simulink model "Control_Loop4_2Model"  (R2013b)
settings: Solver=ode45  StartTime=0.0  StopTime=200  RelTol=1e-3
libraries: commutil2 x756, xpclib x100, etargetslib x98, dspnetwork x98, powerlib_meascontrol x24, commcrc2 x14, dspadpt3 x4, simulink_extras x4, dspmtrx3 x4, simulink x1
(part 1 of 7)
settings Model: Creator=HESL  LastModifiedBy=ANKITA003

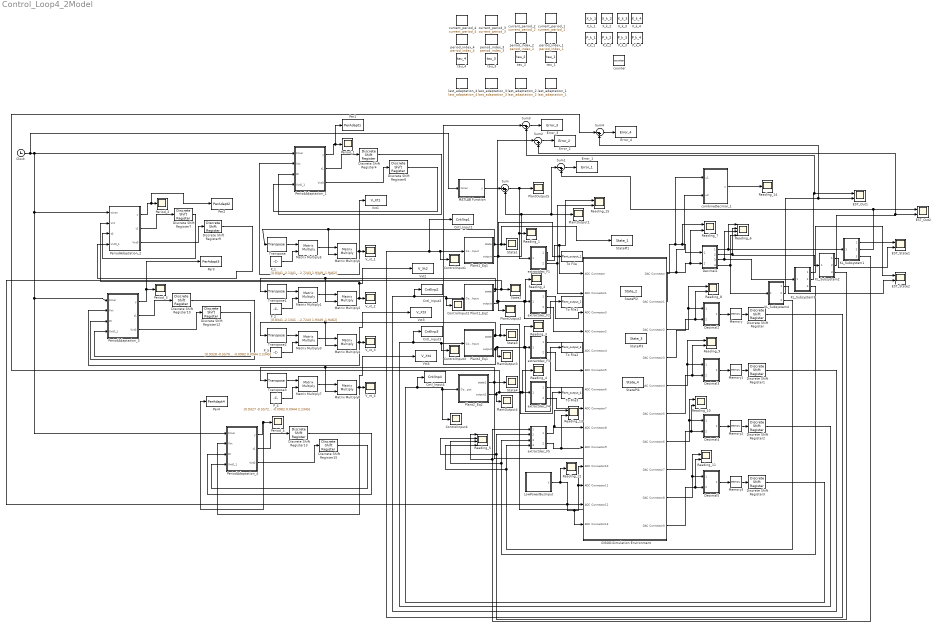
== system Control_Loop4_2Model ==
  Clock : Clock
  Cntl_Input1 : ToFile  Filename=CntlInp1  MatrixName=u
  Cntl_Input2 : ToFile  Filename=CntlInp2  MatrixName=u
  Cntl_Input3 : ToFile  Filename=CntlInp3  MatrixName=u
  Cntl_Input4 : ToFile  Filename=CntlInp4  MatrixName=u
  ControlInput{1..4} (4 alike) : Scope
      ControlInput1 settings: YMin=-4.25  YMax=1.25
      ControlInput2 settings: YMin=-9  YMax=0
      ControlInput3 settings: YMin=-1.60965  YMax=-1.45635  SaveName=ScopeData6
      ControlInput4 settings: YMin=0.01045  YMax=0.01155  SaveName=ScopeData9
  Decimal1 : Subsystem
  Decimal2 : Subsystem
  Decimal3 : Subsystem
  Decimal4 : Subsystem
  Decimal5 : Subsystem
  Discrete Shift Register : powerlib_meascontrol/Additional Components/Discrete Shift Register  NSamples=1  InitialValue=0  Ts=0.150
  Discrete Shift Register1 : powerlib_meascontrol/Additional Components/Discrete Shift Register  NSamples=1  InitialValue=0  Ts=0.150
  Discrete Shift Register{4,6..7,9..10,12..13,15} (8 alike) : powerlib_meascontrol/Additional Components/Discrete Shift Register  NSamples=1  InitialValue=0  Ts=1
  Discrete Shift Register2 : powerlib_meascontrol/Additional Components/Discrete Shift Register  NSamples=1  InitialValue=0  Ts=0.225
  Discrete Shift Register3 : powerlib_meascontrol/Additional Components/Discrete Shift Register  NSamples=1  InitialValue=0  Ts=0.225
  EST_Out1 : Scope  NumInputPorts=2
      settings: YMin=-1.975~-1.92  YMax=-1.55~-1.77  SaveName=ScopeData15
  EST_Out2 : Scope  NumInputPorts=2
      settings: YMin=-4.75e-05~1.71875  YMax=-1e-05~1.71905  SaveName=ScopeData16
  EST_State1 : Scope  NumInputPorts=2
      settings: YMin=-35~-0.1  YMax=40~1.9  SaveName=ScopeData13
  EST_State2 : Scope  NumInputPorts=2
      settings: YMin=-2.5~-0.0003  YMax=1.5~0.001  SaveName=ScopeData14
  Error_1 : ToFile  Filename=Error_1  MatrixName=err_1
  Error_2 : ToFile  Filename=Error_2  MatrixName=err_1
  Error_3 : ToFile  Filename=Error_3  MatrixName=err_1
  Error_4 : ToFile  Filename=Error_4  MatrixName=err_1
  GISOO-Simulation Environment : Subsystem  TreatAsAtomicUnit=on
  KL_Subsystem1 : Subsystem
  KL_Subsystem2 : Subsystem
  KL_Subsystem3 : Subsystem
  KL_Subsystem4 : Subsystem
  LowPowerBusInput : MATLAB Function  TreatAsAtomicUnit=on  SystemSampleTime=0.200
  MATLAB Function : MATLAB Function  TreatAsAtomicUnit=on  SystemSampleTime=0.010
  Matrix Multiply1 : Product  Multiplication=Matrix(*)  SampleTime=0.150
  Matrix Multiply2 : Product  Multiplication=Matrix(*)  SampleTime=0.150
  Matrix Multiply{3..4,7..8} (4 alike) : Product  Multiplication=Matrix(*)  SampleTime=0.225
  Matrix Multiply5 : Product  Multiplication=Matrix(*)  SampleTime=1
  Matrix Multiply6 : Product  Multiplication=Matrix(*)  SampleTime=1
  Memory{,1..3} (4 alike) : Memory
  P_1 : Constant  Value=[0.8341 -2.1341 0.2898 -0.9410;-2.1341 -25.1720 3.5962 -12.7243;0.2898 3.5962 0.5577 1.9349;-0.9410 -12.7243 1.9349 -1.9462]  VectorParams1D=off  SampleTime=1
  P_2 : Constant  Value=[0.8341 -2.1341 0.2898 -0.9410;-2.1341 -25.1720 3.5962 -12.7243;0.2898 3.5962 0.5577 1.9349;-0.9410 -12.7243 1.9349 -1.9462]  VectorParams1D=off  SampleTime=0.150
  P_3 : Constant  Value=[0.9328 -0.5570 0.0394 0.0140;-0.5570 -2.3354 0.2168 -0.0982;0.0394 0.2168 1.0331 0.0944;0.0140 -0.0982 0.0944 2.2345]  VectorParams1D=off  SampleTime=0.225
  P_4 : Constant  Value=[0.9327 -0.5572 0.0394 0.0140;-0.5572 -2.3356 0.2168 -0.0982;0.0394 0.2168 1.0331 0.0944;0.0140 -0.0982 0.0944 2.2345]  VectorParams1D=off  SampleTime=0.225
  P_k_1 : DataStoreMemory  DataStoreName=P_k_1  InitialValue=10*eye(4)  OutDataTypeStr=double
  P_k_2 : DataStoreMemory  DataStoreName=P_k_2  InitialValue=10*eye(4)  OutDataTypeStr=double
  P_k_3 : DataStoreMemory  DataStoreName=P_k_3  InitialValue=10*eye(4)  OutDataTypeStr=double
  P_k_4 : DataStoreMemory  DataStoreName=P_k_4  InitialValue=10*eye(4)  OutDataTypeStr=double
  Per1 : ToFile  Filename=PerAdapt1  MatrixName=P1
  Per2 : ToFile  Filename=PerAdapt2  MatrixName=P2
  Per3 : ToFile  Filename=PerAdapt3  MatrixName=P3
  Per4 : ToFile  Filename=PerAdapt4  MatrixName=P4
  PeriodAdaptation_1 : MATLAB Function  RequirementInfo={} %GIDa_850bbe14_d9da_4034_8937_a8dbb2f822c9  TreatAsAtomicUnit=on  SystemSampleTime=1
  PeriodAdaptation_2 : MATLAB Function  RequirementInfo={} %GIDa_a70684f9_3044_4532_9a1c_a31c50b95e8e  TreatAsAtomicUnit=on  SystemSampleTime=1
  PeriodAdaptation_3 : MATLAB Function  RequirementInfo={} %GIDa_89bb9df0_2bef_4001_9282_b413ac28a927  TreatAsAtomicUnit=on  SystemSampleTime=1
  PeriodAdaptation_4 : MATLAB Function  RequirementInfo={} %GIDa_da02a095_aa0b_4737_8edc_96c2e4425495  TreatAsAtomicUnit=on  SystemSampleTime=1
  Period_{1..4} (4 alike) : Scope
      Period_1 settings: TickLabels=on  YMin=19  YMax=21  SaveName=ScopeData21  SampleInput=on
      Period_2 settings: TickLabels=on  YMin=57  YMax=63  SaveName=ScopeData22  SampleInput=on
      Period_3 settings: TickLabels=on  YMin=15  YMax=15  SaveName=ScopeData23  SampleInput=on
      Period_4 settings: TickLabels=on  YMin=15  YMax=15  SaveName=ScopeData24  SampleInput=on
  Plant1_Eq1 : Subsystem
  Plant1_Eq2 : Subsystem
  Plant2_Eq1 : Subsystem
  Plant2_Eq2 : Subsystem
  PlantOutput{1..5} (5 alike) : Scope
      PlantOutput1 settings: YMin=0.097  YMax=0.117  SaveName=ScopeData4
      PlantOutput2 settings: TimeRange=200  YMin=1.71906  YMax=1.71906  SaveName=ScopeData2
      PlantOutput3 settings: TimeRange=200  YMin=1.7729  YMax=1.7729  SaveName=ScopeData7
      PlantOutput4 settings: YMin=-0.835427  YMax=-0.835427  SaveName=ScopeData10
      PlantOutput5 settings: TimeRange=200  YMin=1.72358  YMax=1.905  SaveName=ScopeData39
  Reading_{1..4,12,14} (6 alike) : Scope
      Reading_1 settings: YMin=1.71875  YMax=1.71935  SaveName=ScopeData25
      Reading_12 settings: YMin=20  YMax=20  SaveName=ScopeData36
      Reading_14 settings: YMin=0  YMax=1.75  SaveName=ScopeData38
      Reading_2 settings: YMin=1.72358  YMax=1.905  SaveName=ScopeData26
      Reading_3 settings: YMin=1.41328  YMax=1.56204  SaveName=ScopeData27
      Reading_4 settings: YMin=1.41328  YMax=1.56204  SaveName=ScopeData28
  Reading_{7..11,13,15} (7 alike) : Scope  NumInputPorts=2
      Reading_10 settings: YMin=1001~2533  YMax=1001~2533  SaveName=ScopeData34
      Reading_11 settings: YMin=1001~3533  YMax=1001~3533  SaveName=ScopeData35
      Reading_13 settings: YMin=1001~0  YMax=1003~3750  SaveName=ScopeData37
      Reading_15 settings: YMin=1~719.057  YMax=1~719.057  SaveName=ScopeData40
      Reading_7 settings: YMin=1~500  YMax=1~4000  SaveName=ScopeData31
      Reading_8 settings: YMin=1003~260  YMax=1003~440  SaveName=ScopeData32
      Reading_9 settings: YMin=950~1187.5  YMax=1050~1312.5  SaveName=ScopeData33
  Reading_5 : Scope  NumInputPorts=4
      settings: YMin=-3.3425~-3.3425~-1.61025~-1.61025  YMax=-3.3225~-3.3225~-1.45689~-1.45689  SaveName=ScopeData29  MaxDataPoints=100000
  Reading_6 : Scope  NumInputPorts=4
      settings: YMin=1.718~1.718~1.4459~1.4459  YMax=1.719~1.719~1.5981~1.5981  SaveName=ScopeData30  MaxDataPoints=100000
  State{1..4} (4 alike) : Scope
      State1 settings: YMin=-0.5  YMax=8  SaveName=ScopeData5
      State2 settings: YMin=0.4  YMax=1  SaveName=ScopeData3
      State3 settings: YMin=0.15  YMax=1.05  SaveName=ScopeData8
      State4 settings: YMin=-0.055  YMax=-0.042  SaveName=ScopeData12
  StatePl1 : ToFile  Filename=State_1  MatrixName=x
  StatePl2 : ToFile  Filename=State_2  MatrixName=x
  StatePl3 : ToFile  Filename=State_3  MatrixName=x
  StatePl4 : ToFile  Filename=State_4  MatrixName=x
  Sum : Sum  Inputs=|++
  Sum{1..4} (4 alike) : Sum  Inputs=|-+  SampleTime=1
  To File : ToFile  Filename=Plant_output_1  MatrixName=Out
  To File1 : ToFile  Filename=Plant_output_2  MatrixName=Out
  To File2 : ToFile  Filename=Plant_output_3  MatrixName=Out
  To File3 : ToFile  Filename=Plant_output_4  MatrixName=Out
  Transpose{,1..3} (4 alike) : dspmtrx3/Transpose  Hermitian=off  overflowFlag=off
  V_xt_{1..4} (4 alike) : Scope
      V_xt_1 settings: TickLabels=on  YMin=-0.19  YMax=-0.085  SaveName=ScopeData17  SampleInput=on
      V_xt_2 settings: TickLabels=on  YMin=-2.5e-06  YMax=4.5e-05  SaveName=ScopeData18  SampleInput=on
      V_xt_3 settings: TickLabels=on  YMin=0.0031225  YMax=0.003133  SaveName=ScopeData19  SampleInput=on
      V_xt_4 settings: TickLabels=on  YMin=0.00322  YMax=0.00322002  SaveName=ScopeData20  SampleInput=on
  Vxt1 : ToFile  Filename=V_Xt1  MatrixName=Vxt
  Vxt2 : ToFile  Filename=V_Xt2  MatrixName=Vxt
  Vxt3 : ToFile  Filename=V_Xt3  MatrixName=Vxt
  Vxt4 : ToFile  Filename=V_Xt4  MatrixName=Vxt
  X_k_1 : DataStoreMemory  DataStoreName=X_k_1  InitialValue=zeros(4,1)  OutDataTypeStr=double
  X_k_2 : DataStoreMemory  DataStoreName=X_k_2  InitialValue=zeros(4,1)  OutDataTypeStr=double
  X_k_3 : DataStoreMemory  DataStoreName=X_k_3  InitialValue=zeros(4,1)  OutDataTypeStr=double
  X_k_4 : DataStoreMemory  DataStoreName=X_k_4  InitialValue=zeros(4,1)  OutDataTypeStr=double
  combineDecimal_1 : MATLAB Function  TreatAsAtomicUnit=on  SystemSampleTime=0.010
  counter : DataStoreMemory  DataStoreName=counter  OutDataTypeStr=double
  current_period_1 : DataStoreMemory  DataStoreName=current_period_1  InitialValue=10  OutDataTypeStr=double
  current_period_2 : DataStoreMemory  DataStoreName=current_period_2  InitialValue=10  OutDataTypeStr=double
  current_period_3 : DataStoreMemory  DataStoreName=current_period_3  InitialValue=15  OutDataTypeStr=double
  current_period_4 : DataStoreMemory  DataStoreName=current_period_4  InitialValue=15  OutDataTypeStr=double
  extractdec_F1 : Subsystem
  extractdec_F2 : Subsystem
  extractdec_F3 : Subsystem
  extractdec_F4 : Subsystem
  extractdec_F5 : Subsystem
  last_adaptation_1 : DataStoreMemory  DataStoreName=last_adaptation_1  OutDataTypeStr=double
  last_adaptation_2 : DataStoreMemory  DataStoreName=last_adaptation_2  OutDataTypeStr=double
  last_adaptation_3 : DataStoreMemory  DataStoreName=last_adaptation_3  OutDataTypeStr=double
  last_adaptation_4 : DataStoreMemory  DataStoreName=last_adaptation_4  OutDataTypeStr=double
  period_index_1 : DataStoreMemory  DataStoreName=period_index_1  InitialValue=1  OutDataTypeStr=double
  period_index_2 : DataStoreMemory  DataStoreName=period_index_2  InitialValue=1  OutDataTypeStr=double
  period_index_3 : DataStoreMemory  DataStoreName=period_index_3  InitialValue=1  OutDataTypeStr=double
  period_index_4 : DataStoreMemory  DataStoreName=period_index_4  InitialValue=1  OutDataTypeStr=double
  tau_1 : DataStoreMemory  DataStoreName=tau_1  OutDataTypeStr=double
  tau_2 : DataStoreMemory  DataStoreName=tau_2  OutDataTypeStr=double
  tau_3 : DataStoreMemory  DataStoreName=tau_3  OutDataTypeStr=double
  tau_4 : DataStoreMemory  DataStoreName=tau_4  OutDataTypeStr=double
  wires:
  Plant2_Eq1/2(output) -> To File2/1, extractdec_F3/1(In1), Reading_3/1, PlantOutput3/1, Sum3/1
  extractdec_F1/1(Out1) -> Reading_15/1, GISOO-Simulation Environment/1(ADC Connector)
  extractdec_F1/2(Out2) -> GISOO-Simulation Environment/2(ADC Connector1), Reading_15/2
  extractdec_F2/1(Out1) -> GISOO-Simulation Environment/3(ADC Connector3)
  extractdec_F2/2(Out2) -> GISOO-Simulation Environment/4(ADC Connector2)
  extractdec_F3/1(Out1) -> GISOO-Simulation Environment/5(ADC Connector4)
  extractdec_F3/2(Out2) -> GISOO-Simulation Environment/6(ADC Connector5)
  extractdec_F4/1(Out1) -> GISOO-Simulation Environment/7(ADC Connector6)
  extractdec_F4/2(Out2) -> GISOO-Simulation Environment/8(ADC Connector7)
  extractdec_F5/1(Out1) -> Reading_13/1, GISOO-Simulation Environment/9(ADC Connector8)
  extractdec_F5/2(Out2) -> Reading_13/2, GISOO-Simulation Environment/10(ADC Connector9)
  LowPowerBusInput/1(y) -> Reading_12/1, GISOO-Simulation Environment/14(ADC Connector13), GISOO-Simulation Environment/11(ADC Connector10), GISOO-Simulation Environment/12(ADC Connector11), GISOO-Simulation Environment/13(ADC Connector12)
  GISOO-Simulation Environment/1(DAC Connector) -> combineDecimal_1/1(u1), Reading_7/1, Decimal1/1(In1)
  GISOO-Simulation Environment/4(DAC Connector3) -> Reading_8/2, Decimal2/2(In2)
  GISOO-Simulation Environment/3(DAC Connector2) -> Reading_8/1, Decimal2/1(In1)
  GISOO-Simulation Environment/5(DAC Connector4) -> Reading_9/1, Decimal3/1(In1)
  GISOO-Simulation Environment/6(DAC Connector5) -> Reading_9/2, Decimal3/2(In2)
  GISOO-Simulation Environment/7(DAC Connector6) -> Reading_10/1, Decimal4/1(In1)
  GISOO-Simulation Environment/8(DAC Connector7) -> Reading_10/2, Decimal4/2(In2)
  GISOO-Simulation Environment/9(DAC Connector8) -> Reading_11/1, Decimal5/1(In1)
  GISOO-Simulation Environment/10(DAC Connector9) -> Reading_11/2, Decimal5/2(In2)
  Decimal1/1(Out1) -> KL_Subsystem1/1(In1), Reading_6/1
  Decimal1/2(Out2) -> KL_Subsystem2/1(In1), Reading_6/2
  Decimal1/3(Out3) -> Reading_6/3, KL_Subsystem3/1(In1)
  Decimal1/4(Out4) -> KL_Subsystem4/1(In1), Reading_6/4
  Discrete Shift Register/1 -> Cntl_Input1/1, Plant1_Eq1/1(ControlInput), ControlInput1/1
  Discrete Shift Register1/1 -> Cntl_Input2/1, ControlInput2/1, Plant1_Eq2/1(ControlInput)
  Discrete Shift Register2/1 -> ControlInput3/1, Plant2_Eq1/1(ControlInput), Cntl_Input3/1
  Decimal2/1(Out1) -> Memory/1
  Memory/1 -> Discrete Shift Register/1
  Decimal3/1(Out1) -> Memory1/1
  Memory1/1 -> Discrete Shift Register1/1
  Decimal4/1(Out1) -> Memory2/1
  Memory2/1 -> Discrete Shift Register2/1
  Decimal5/1(Out1) -> Memory3/1
  Memory3/1 -> Discrete Shift Register3/1
  KL_Subsystem1/3(Out3) -> Reading_5/1, extractdec_F5/1(In1)
  KL_Subsystem2/3(Out3) -> Reading_5/2, extractdec_F5/2(In2)
  KL_Subsystem3/3(Out3) -> Reading_5/3, extractdec_F5/3(In3)
  KL_Subsystem4/3(Out3) -> Reading_5/4, extractdec_F5/4(In4)
  KL_Subsystem1/1(Out1) -> EST_State1/1
  KL_Subsystem2/1(Out1) -> EST_State1/2
  KL_Subsystem3/1(Out1) -> EST_State2/1
  KL_Subsystem4/1(Out1) -> EST_State2/2
  KL_Subsystem4/2(Out2) -> EST_Out1/2, Sum4/2
  Transpose/1 -> Matrix Multiply5/1
  Matrix Multiply5/1 -> Matrix Multiply6/1
  P_1/1 -> Matrix Multiply5/2
  Plant1_Eq1/1(state) -> Matrix Multiply6/2, Transpose/1, StatePl1/1, State1/1
  Transpose1/1 -> Matrix Multiply1/1
  Matrix Multiply1/1 -> Matrix Multiply2/1
  P_2/1 -> Matrix Multiply1/2
  Plant1_Eq2/1(state) -> Matrix Multiply2/2, Transpose1/1, StatePl2/1, State2/1
  Transpose2/1 -> Matrix Multiply3/1
  Matrix Multiply3/1 -> Matrix Multiply4/1
  P_3/1 -> Matrix Multiply3/2
  Plant2_Eq1/1(state) -> Matrix Multiply4/2, Transpose2/1, StatePl3/1, State3/1
  Transpose3/1 -> Matrix Multiply7/1
  Matrix Multiply7/1 -> Matrix Multiply8/1
  P_4/1 -> Matrix Multiply7/2
  Plant2_Eq2/1(state1) -> StatePl4/1, State4/1, Matrix Multiply8/2, Transpose3/1
  Matrix Multiply6/1 -> Vxt1/1, PeriodAdaptation_1/2(Vxt), V_xt_1/1
  PeriodAdaptation_1/2(t1) -> Discrete Shift Register4/1
  Discrete Shift Register4/1 -> PeriodAdaptation_1/3(t0)
  PeriodAdaptation_1/3(Vxt0) -> Discrete Shift Register6/1
  Discrete Shift Register6/1 -> PeriodAdaptation_1/4(Vxt0_1)
  PeriodAdaptation_1/1(y) -> Per1/1, Period_1/1
  Matrix Multiply2/1 -> Vxt2/1, PeriodAdaptation_2/2(Vxt), V_xt_2/1
  PeriodAdaptation_2/2(t1) -> Discrete Shift Register7/1
  Discrete Shift Register7/1 -> PeriodAdaptation_2/3(t0)
  PeriodAdaptation_2/3(Vxt0) -> Discrete Shift Register9/1
  Discrete Shift Register9/1 -> PeriodAdaptation_2/4(Vxt0_1)
  PeriodAdaptation_2/1(y) -> Per2/1, Period_2/1
  Matrix Multiply4/1 -> PeriodAdaptation_3/2(Vxt), Vxt3/1, V_xt_3/1
  PeriodAdaptation_3/2(t1) -> Discrete Shift Register10/1
  Discrete Shift Register10/1 -> PeriodAdaptation_3/3(t0)
  PeriodAdaptation_3/3(Vxt0) -> Discrete Shift Register12/1
  Discrete Shift Register12/1 -> PeriodAdaptation_3/4(Vxt0_1)
  PeriodAdaptation_3/1(y) -> Per3/1, Period_3/1
  Matrix Multiply8/1 -> PeriodAdaptation_4/2(Vxt), Vxt4/1, V_xt_4/1
  PeriodAdaptation_4/2(t1) -> Discrete Shift Register13/1
  Discrete Shift Register13/1 -> PeriodAdaptation_4/3(t0)
  PeriodAdaptation_4/3(Vxt0) -> Discrete Shift Register15/1
  Discrete Shift Register15/1 -> PeriodAdaptation_4/4(Vxt0_1)
  PeriodAdaptation_4/1(y) -> Per4/1, Period_4/1
  Clock/1 -> MATLAB Function/1(timer), PeriodAdaptation_4/1(timer), PeriodAdaptation_3/1(timer), PeriodAdaptation_2/1(timer), PeriodAdaptation_1/1(timer)
  Plant1_Eq1/2(output) -> To File/1, Sum1/1, PlantOutput1/1, Sum/2
  GISOO-Simulation Environment/2(DAC Connector1) -> combineDecimal_1/2(u2), Reading_7/2, Decimal1/2(In2)
  combineDecimal_1/1(y) -> Reading_14/1
  MATLAB Function/1(y) -> Sum/1
  Sum/1 -> Reading_1/1, extractdec_F1/1(In1), PlantOutput5/1
  KL_Subsystem1/2(Out2) -> Sum1/2, EST_Out2/1
  Sum1/1 -> Error_1/1
  Sum2/1 -> Error_2/1
  Sum3/1 -> Error_3/1
  Sum4/1 -> Error_4/1
  Plant1_Eq2/2(output) -> To File1/1, Reading_2/1, extractdec_F2/1(In1), PlantOutput2/1, Sum2/1
  KL_Subsystem2/2(Out2) -> EST_Out2/2, Sum2/2
  KL_Subsystem3/2(Out2) -> EST_Out1/1, Sum3/2
  Plant2_Eq2/2(output1) -> PlantOutput4/1, Sum4/1, To File3/1, Reading_4/1, extractdec_F4/1(In1)
  Discrete Shift Register3/1 -> Cntl_Input4/1, ControlInput4/1, Plant2_Eq2/1(ControlInput)

== system Control_Loop4_2Model/Decimal1 ==
  In1 : Inport
  In2 : Inport  Port=2
  Discrete Shift Register{,1..3} (4 alike) : powerlib_meascontrol/Additional Components/Discrete Shift Register  NSamples=1  InitialValue=0  Ts=0.010
  combineDecimal_1 : MATLAB Function  TreatAsAtomicUnit=on  SystemSampleTime=0.010
  Out1 : Outport
  Out2 : Outport  Port=2
  Out3 : Outport  Port=3
  Out4 : Outport  Port=4
  wires:
  combineDecimal_1/1(y1) -> Out1/1
  In2/1 -> combineDecimal_1/2(u2)
  In1/1 -> combineDecimal_1/1(u1)
  combineDecimal_1/5(x1) -> Discrete Shift Register/1
  combineDecimal_1/6(x2) -> Discrete Shift Register1/1
  combineDecimal_1/7(x3) -> Discrete Shift Register2/1
  combineDecimal_1/8(x4) -> Discrete Shift Register3/1
  Discrete Shift Register3/1 -> combineDecimal_1/6(x4_prev)
  Discrete Shift Register2/1 -> combineDecimal_1/5(x3_prev)
  Discrete Shift Register1/1 -> combineDecimal_1/4(x2_prev)
  Discrete Shift Register/1 -> combineDecimal_1/3(x1_prev)
  combineDecimal_1/2(y2) -> Out2/1
  combineDecimal_1/3(y3) -> Out3/1
  combineDecimal_1/4(y4) -> Out4/1

== system Control_Loop4_2Model/Decimal2 ==
  In1 : Inport
  In2 : Inport  Port=2
  Scope : Scope
      settings: YMin=-5.964  YMax=-5.396  SaveName=ScopeData11
  combineDecimal_1 : MATLAB Function  TreatAsAtomicUnit=on  SystemSampleTime=0.010
  Out1 : Outport
  wires:
  combineDecimal_1/1(y) -> Scope/1, Out1/1
  In2/1 -> combineDecimal_1/2(u2)
  In1/1 -> combineDecimal_1/1(u1)

== system Control_Loop4_2Model/Decimal3 ==
  In1 : Inport
  In2 : Inport  Port=2
  Scope : Scope
      settings: YMin=-5.964  YMax=-5.396  SaveName=ScopeData11
  combineDecimal_1 : MATLAB Function  TreatAsAtomicUnit=on  SystemSampleTime=0.010
  Out1 : Outport
  wires:
  combineDecimal_1/1(y) -> Scope/1, Out1/1
  In2/1 -> combineDecimal_1/2(u2)
  In1/1 -> combineDecimal_1/1(u1)

== system Control_Loop4_2Model/Decimal4 ==
  In1 : Inport
  In2 : Inport  Port=2
  Scope : Scope
      settings: YMin=-5.964  YMax=-5.396  SaveName=ScopeData11
  combineDecimal_1 : MATLAB Function  TreatAsAtomicUnit=on  SystemSampleTime=0.010
  Out1 : Outport
  wires:
  combineDecimal_1/1(y) -> Scope/1, Out1/1
  In2/1 -> combineDecimal_1/2(u2)
  In1/1 -> combineDecimal_1/1(u1)

== system Control_Loop4_2Model/Decimal5 ==
  In1 : Inport
  In2 : Inport  Port=2
  Scope : Scope
      settings: YMin=-5.964  YMax=-5.396  SaveName=ScopeData11
  combineDecimal_1 : MATLAB Function  TreatAsAtomicUnit=on  SystemSampleTime=0.010
  Out1 : Outport
  wires:
  combineDecimal_1/1(y) -> Scope/1, Out1/1
  In2/1 -> combineDecimal_1/2(u2)
  In1/1 -> combineDecimal_1/1(u1)

== system Control_Loop4_2Model/GISOO-Simulation Environment ==
  ADC Connector : Inport
  ADC Connector1 : Inport  Port=2
  ADC Connector3 : Inport  Port=3
  ADC Connector2 : Inport  Port=4
  ADC Connector4 : Inport  Port=5
  ADC Connector5 : Inport  Port=6
  ADC Connector6 : Inport  Port=7
  ADC Connector7 : Inport  Port=8
  ADC Connector8 : Inport  Port=9
  ADC Connector9 : Inport  Port=10
  ADC Connector10 : Inport  Port=11
  ADC Connector11 : Inport  Port=12
  ADC Connector12 : Inport  Port=13
  ADC Connector13 : Inport  Port=14
  CoojaConnector : Subsystem
  SkyMote : Subsystem  mask{moteID=1, PacketType=6}
      mask prompts: PacketType "Serial Packet Type (Required block receives Serial data):"
  SkyMote1 : Subsystem  mask{moteID=5, PacketType=6}
      mask prompts: PacketType "Serial Packet Type (Required block receives Serial data):"
  SkyMote10 : Subsystem  mask{moteID=19, PacketType=6}
      mask prompts: PacketType "Serial Packet Type (Required block receives Serial data):"
  SkyMote11 : Subsystem  mask{moteID=20, PacketType=6}
      mask prompts: PacketType "Serial Packet Type (Required block receives Serial data):"
  SkyMote12 : Subsystem  mask{moteID=21, PacketType=6}
      mask prompts: PacketType "Serial Packet Type (Required block receives Serial data):"
  SkyMote13 : Subsystem  mask{moteID=22, PacketType=6}
      mask prompts: PacketType "Serial Packet Type (Required block receives Serial data):"
  SkyMote2 : Subsystem  mask{moteID=2, PacketType=6}
      mask prompts: PacketType "Serial Packet Type (Required block receives Serial data):"
  SkyMote3 : Subsystem  mask{moteID=7, PacketType=6}
      mask prompts: PacketType "Serial Packet Type (Required block receives Serial data):"
  SkyMote4 : Subsystem  mask{moteID=3, PacketType=6}
      mask prompts: PacketType "Serial Packet Type (Required block receives Serial data):"
  SkyMote5 : Subsystem  mask{moteID=4, PacketType=6}
      mask prompts: PacketType "Serial Packet Type (Required block receives Serial data):"
  SkyMote6 : Subsystem  mask{moteID=6, PacketType=6}
      mask prompts: PacketType "Serial Packet Type (Required block receives Serial data):"
  SkyMote7 : Subsystem  mask{moteID=9, PacketType=6}
      mask prompts: PacketType "Serial Packet Type (Required block receives Serial data):"
  SkyMote8 : Subsystem  mask{moteID=8, PacketType=6}
      mask prompts: PacketType "Serial Packet Type (Required block receives Serial data):"
  SkyMote9 : Subsystem  mask{moteID=10, PacketType=6}
      mask prompts: PacketType "Serial Packet Type (Required block receives Serial data):"
  SynchronizerLoop : WhileIterator  MaxIters=-1  WhileBlockType=do-while  ShowIterationPort=on
  DAC Connector : Outport
  DAC Connector1 : Outport  Port=2
  DAC Connector2 : Outport  Port=3
  DAC Connector3 : Outport  Port=4
  DAC Connector4 : Outport  Port=5
  DAC Connector5 : Outport  Port=6
  DAC Connector6 : Outport  Port=7
  DAC Connector7 : Outport  Port=8
  DAC Connector8 : Outport  Port=9
  DAC Connector9 : Outport  Port=10
  wires:
  SynchronizerLoop/1 -> CoojaConnector/1(DelayNum.)
  CoojaConnector/1(Wait) -> SynchronizerLoop/1
  ADC Connector/1 -> SkyMote/1(ADC0)
  ADC Connector1/1 -> SkyMote/2(ADC1)
  SkyMote1/1(DAC0) -> DAC Connector/1
  SkyMote1/2(DAC1) -> DAC Connector1/1
  SkyMote3/1(DAC0) -> DAC Connector2/1
  SkyMote3/2(DAC1) -> DAC Connector3/1
  ADC Connector3/1 -> SkyMote2/1(ADC0)
  ADC Connector2/1 -> SkyMote2/2(ADC1)
  ADC Connector4/1 -> SkyMote4/1(ADC0)
  ADC Connector5/1 -> SkyMote4/2(ADC1)
  ADC Connector6/1 -> SkyMote5/1(ADC0)
  ADC Connector7/1 -> SkyMote5/2(ADC1)
  ADC Connector8/1 -> SkyMote6/1(ADC0)
  ADC Connector9/1 -> SkyMote6/2(ADC1)
  SkyMote8/1(DAC0) -> DAC Connector4/1
  SkyMote8/2(DAC1) -> DAC Connector5/1
  SkyMote7/1(DAC0) -> DAC Connector6/1
  SkyMote7/2(DAC1) -> DAC Connector7/1
  SkyMote9/1(DAC0) -> DAC Connector8/1
  SkyMote9/2(DAC1) -> DAC Connector9/1
  ADC Connector10/1 -> SkyMote10/1(ADC0)
  ADC Connector11/1 -> SkyMote11/1(ADC0)
  ADC Connector12/1 -> SkyMote12/1(ADC0)
  ADC Connector13/1 -> SkyMote13/1(ADC0)

== system Control_Loop4_2Model/KL_Subsystem1 ==
  In1 : Inport
  Constant : Constant  Value=[-1.9393 -13.1373 0.0842 -13.0264]  VectorParams1D=off  SampleTime=0.150
  Constant1 : Constant  Value=[0.001093;0.01368;-0.0009885;-0.01235]  VectorParams1D=off  SampleTime=0.150
  Discrete Shift Register2 : powerlib_meascontrol/Additional Components/Discrete Shift Register  NSamples=1  InitialValue=0  Ts=0.150
  Discrete Shift Register3 : powerlib_meascontrol/Additional Components/Discrete Shift Register  NSamples=1  InitialValue=0  Ts=1
  Kalman Filter : dspadpt3/Kalman Filter  num_targets=1  sourceEnable=Always  isReset=on  X=zeros([4, 1])  P=10*eye(4)  A="[1    0.1336  0.004942   0.01014;0    0.7947   0.06174    0.1284;0   0.01483     0.995    0.1398;0    0.1852  -0.06248    0.8701]"  sourceMeasure=Specify via Dialog  H=[1 0 0 0]  Q=0.5*eye(4)  R=0.8  isOutputEstMeasure=on  isOutputEstState=on  isOutputEstError=off  isOutputPrdMeasure=on  isOutputPrdState=on  isOutputPrdError=off
  Matrix Multiply : Product  Multiplication=Matrix(*)  SampleTime=0.150
  Matrix Multiply1 : Product  Multiplication=Matrix(*)  SampleTime=0.150
  Memory2 : Memory
  Rate Transition : RateTransition  OutPortSampleTime=0.150
  Sum : Sum  Inputs=|++
  Out1 : Outport
  Out2 : Outport  Port=2
  Out3 : Outport  Port=3
  wires:
  Kalman Filter/3 -> Out2/1
  In1/1 -> Rate Transition/1
  Sum/1 -> Out1/1, Matrix Multiply/2
  Matrix Multiply/1 -> Memory2/1
  Discrete Shift Register2/1 -> Discrete Shift Register3/1, Matrix Multiply1/2
  Constant/1 -> Matrix Multiply/1
  Kalman Filter/4 -> Sum/1
  Constant1/1 -> Matrix Multiply1/1
  Matrix Multiply1/1 -> Sum/2
  Rate Transition/1 -> Kalman Filter/1
  Memory2/1 -> Discrete Shift Register2/1
  Discrete Shift Register3/1 -> Out3/1

== system Control_Loop4_2Model/KL_Subsystem2 ==
  In1 : Inport
  Constant1 : Constant  Value=[-1.9393 -13.1373 0.0842 -13.0264]  VectorParams1D=off  SampleTime=0.150
  Constant2 : Constant  Value=[0.001093;0.01368;-0.0009885;-0.01235]  VectorParams1D=off  SampleTime=0.150
  Discrete Shift Register2 : powerlib_meascontrol/Additional Components/Discrete Shift Register  NSamples=1  InitialValue=0  Ts=0.150
  Discrete Shift Register3 : powerlib_meascontrol/Additional Components/Discrete Shift Register  NSamples=1  InitialValue=0  Ts=1
  Kalman Filter1 : dspadpt3/Kalman Filter  num_targets=1  sourceEnable=Always  isReset=on  X=zeros([4, 1])  P=10*eye(4)  A="[1    0.1336  0.004942   0.01014;0    0.7947   0.06174    0.1284;0   0.01483     0.995    0.1398;0    0.1852  -0.06248    0.8701]"  sourceMeasure=Specify via Dialog  H=[1 0 0 0]  Q=0.5*eye(4)  R=0.8  isOutputEstMeasure=on  isOutputEstState=on  isOutputEstError=off  isOutputPrdMeasure=on  isOutputPrdState=on  isOutputPrdError=off
  Matrix Multiply1 : Product  Multiplication=Matrix(*)  SampleTime=0.150
  Matrix Multiply2 : Product  Multiplication=Matrix(*)  SampleTime=0.150
  Memory2 : Memory
  Rate Transition : RateTransition  OutPortSampleTime=0.150
  Sum : Sum  Inputs=|++
  Out1 : Outport
  Out2 : Outport  Port=2
  Out3 : Outport  Port=3
  wires:
  Kalman Filter1/3 -> Out2/1
  In1/1 -> Rate Transition/1
  Sum/1 -> Out1/1, Matrix Multiply1/2
  Matrix Multiply1/1 -> Memory2/1
  Discrete Shift Register2/1 -> Discrete Shift Register3/1, Matrix Multiply2/2
  Constant1/1 -> Matrix Multiply1/1
  Kalman Filter1/4 -> Sum/1
  Constant2/1 -> Matrix Multiply2/1
  Matrix Multiply2/1 -> Sum/2
  Rate Transition/1 -> Kalman Filter1/1
  Discrete Shift Register3/1 -> Out3/1

== system Control_Loop4_2Model/KL_Subsystem3 ==
  In1 : Inport
  Constant1 : Constant  Value=[-1.0076 -0.6317 -0.1954 -0.3814]  VectorParams1D=off  SampleTime=0.230
  Constant2 : Constant  Value=[0.00541;0.04305;-0.004007;-0.03165]  VectorParams1D=off  SampleTime=0.230
  Discrete Shift Register2 : powerlib_meascontrol/Additional Components/Discrete Shift Register  NSamples=1  InitialValue=0  Ts=0.230
  Discrete Shift Register3 : powerlib_meascontrol/Additional Components/Discrete Shift Register  NSamples=1  InitialValue=0  Ts=1
  Kalman Filter1 : dspadpt3/Kalman Filter  num_targets=1  sourceEnable=Always  isReset=on  X=zeros([4, 1])  P=10*eye(4)  A="[1    0.1709  0.008014   0.01266;0    0.5696    0.0633     0.103;0   0.04007    0.9916    0.2117;0    0.3165  -0.06864    0.8886]"  sourceMeasure=Specify via Dialog  H=[1 0 0 0]  Q=0.5*eye(4)  R=0.8  isOutputEstMeasure=on  isOutputEstState=on  isOutputEstError=off  isOutputPrdMeasure=on  isOutputPrdState=on  isOutputPrdError=off
  Matrix Multiply1 : Product  Multiplication=Matrix(*)  SampleTime=0.230
  Matrix Multiply2 : Product  Multiplication=Matrix(*)  SampleTime=0.230
  Memory2 : Memory
  Rate Transition : RateTransition  OutPortSampleTime=0.230
  Sum : Sum  Inputs=|++
  Out1 : Outport
  Out2 : Outport  Port=2
  Out3 : Outport  Port=3
  wires:
  Kalman Filter1/3 -> Out2/1
  In1/1 -> Rate Transition/1
  Sum/1 -> Out1/1, Matrix Multiply1/2
  Matrix Multiply1/1 -> Memory2/1
  Discrete Shift Register2/1 -> Discrete Shift Register3/1, Matrix Multiply2/2
  Constant1/1 -> Matrix Multiply1/1
  Kalman Filter1/4 -> Sum/1
  Constant2/1 -> Matrix Multiply2/1
  Matrix Multiply2/1 -> Sum/2
  Rate Transition/1 -> Kalman Filter1/1
  Discrete Shift Register3/1 -> Out3/1
  Memory2/1 -> Discrete Shift Register2/1

== system Control_Loop4_2Model/KL_Subsystem4 ==
  In1 : Inport
  Constant : Constant  Value=[-1.0076 -0.6317 -0.1954 -0.3814]  VectorParams1D=off  SampleTime=0.230
  Constant1 : Constant  Value=[0.00541;0.04305;-0.004007;-0.03165]  VectorParams1D=off  SampleTime=0.230
  Discrete Shift Register1 : powerlib_meascontrol/Additional Components/Discrete Shift Register  NSamples=1  InitialValue=0  Ts=0.230
  Discrete Shift Register3 : powerlib_meascontrol/Additional Components/Discrete Shift Register  NSamples=1  InitialValue=0  Ts=1
  Kalman Filter : dspadpt3/Kalman Filter  num_targets=1  sourceEnable=Always  isReset=on  X=zeros([4, 1])  P=10*eye(4)  A=[1 0.1709 0.008014 0.01266;0 0.5696 0.0633 0.103;0 0.04007 0.9916 0.2117;0 0.3165 -0.06864 0.8886]  sourceMeasure=Specify via Dialog  H=[1 0 0 0]  Q=0.05*eye(4)  R=0.8  isOutputEstMeasure=on  isOutputEstState=on  isOutputEstError=off  isOutputPrdMeasure=on  isOutputPrdState=on  isOutputPrdError=off
  Matrix Multiply : Product  Multiplication=Matrix(*)  SampleTime=0.230
  Matrix Multiply1 : Product  Multiplication=Matrix(*)  SampleTime=0.230
  Memory1 : Memory
  Rate Transition : RateTransition  OutPortSampleTime=0.230
  Sum : Sum  Inputs=|++
  Out1 : Outport
  Out2 : Outport  Port=2
  Out3 : Outport  Port=3
  wires:
  Kalman Filter/3 -> Out2/1
  In1/1 -> Rate Transition/1
  Matrix Multiply/1 -> Memory1/1
  Memory1/1 -> Discrete Shift Register1/1
  Constant/1 -> Matrix Multiply/1
  Kalman Filter/4 -> Sum/1
  Constant1/1 -> Matrix Multiply1/1
  Matrix Multiply1/1 -> Sum/2
  Sum/1 -> Out1/1, Matrix Multiply/2
  Rate Transition/1 -> Kalman Filter/1
  Discrete Shift Register1/1 -> Matrix Multiply1/2, Discrete Shift Register3/1
  Discrete Shift Register3/1 -> Out3/1

== system Control_Loop4_2Model/Plant1_Eq1 ==
  ControlInput : Inport  SampleTime=1
  Constant : Constant  Value=[1 0 0 0]  VectorParams1D=off  SampleTime=0.010
  Constant1 : Constant  Value=[-0.05;-0.05;-0.05;-0.05]  VectorParams1D=off  SampleTime=0.010
  Matrix Multiply6 : Product  Multiplication=Matrix(*)  SampleTime=0.010
  State-Space (with initial outputs) : simulink_extras/Additional Linear/State-Space (with initial outputs)  A=[0 1.0000 0 0;0 -1.6500 0.5000 1.0000;0 0 0 1.0000;0 1.5000 -0.5000 -1.0000]  B=[0;0.1100;0;-0.1000]  C=[1 0 0 0;0 1 0 0;0 0 1 0;0 0 0 1]  D=[0;0;0;0]  U0=0  Y0=1
  State1 : Scope
      settings: YMin=-0.5  YMax=1.1  SaveName=ScopeData41
  State2 : Scope
      settings: YMin=-0.07  YMax=0.08  SaveName=ScopeData42
  Sum : Sum  Inputs=|++
  state : Outport  SampleTime=1
  output : Outport  Port=2  SampleTime=1
  wires:
  State-Space (with initial outputs)/1 -> Sum/1, Matrix Multiply6/2
  Constant/1 -> Matrix Multiply6/1
  ControlInput/1 -> State-Space (with initial outputs)/1
  Sum/1 -> State2/1, state/1
  Constant1/1 -> Sum/2
  Matrix Multiply6/1 -> State1/1, output/1

== system Control_Loop4_2Model/Plant1_Eq2 ==
  ControlInput : Inport  SampleTime=1
  Constant : Constant  Value=[1 0 0 0]  VectorParams1D=off  SampleTime=0.010
  Constant1 : Constant  Value=[-0.05;-0.05;-0.05;-0.05]  VectorParams1D=off  SampleTime=0.010
  Matrix Multiply6 : Product  Multiplication=Matrix(*)  SampleTime=0.010
  State-Space (with initial outputs) : simulink_extras/Additional Linear/State-Space (with initial outputs)  A=[0 1.0000 0 0;0 -1.6500 0.5000 1.0000;0 0 0 1.0000;0 1.5000 -0.5000 -1.0000]  B=[0;0.1100;0;-0.1000]  C=[1 0 0 0;0 1 0 0;0 0 1 0;0 0 0 1]  D=[0;0;0;0]  U0=0  Y0=1
  State1 : Scope
      settings: YMin=-0.5  YMax=1.1  SaveName=ScopeData43
  State2 : Scope
      settings: YMin=-0.07  YMax=0.08  SaveName=ScopeData44
  Sum : Sum  Inputs=|++
  state : Outport  SampleTime=1
  output : Outport  Port=2  SampleTime=1
  wires:
  State-Space (with initial outputs)/1 -> Sum/1, Matrix Multiply6/2
  Constant/1 -> Matrix Multiply6/1
  ControlInput/1 -> State-Space (with initial outputs)/1
  Sum/1 -> state/1, State2/1
  Constant1/1 -> Sum/2
  Matrix Multiply6/1 -> output/1, State1/1

== system Control_Loop4_2Model/Plant2_Eq1 ==
  ControlInput : Inport  SampleTime=1
  Constant1 : Constant  Value=[1 0 0 0]  VectorParams1D=off  SampleTime=0.010
  Constant2 : Constant  Value=[-0.05;-0.05;-0.05;-0.05]  VectorParams1D=off  SampleTime=0.010
  Matrix Multiply4 : Product  Multiplication=Matrix(*)  SampleTime=0.010
  State-Space (with initial outputs) : simulink_extras/Additional Linear/State-Space (with initial outputs)  A=[0 1.0000 0 0;0 -2.6667 0.4000 0.6000;0 0 0 1.0000;0 2.0000 -0.4000 -0.6000]  B=[0;0.2667;0;-0.2000]  C=[1 0 0 0;0 1 0 0;0 0 1 0;0 0 0 1]  D=[0;0;0;0]  U0=0  Y0=1
  State3 : Scope
      settings: YMin=-0.5  YMax=1.1  SaveName=ScopeData47
  State4 : Scope
      settings: YMin=-0.07  YMax=0.08  SaveName=ScopeData48
  Sum3 : Sum  Inputs=|++
  state : Outport  SampleTime=1
  output : Outport  Port=2  SampleTime=1
  wires:
  State-Space (with initial outputs)/1 -> Sum3/1, Matrix Multiply4/2
  Constant1/1 -> Matrix Multiply4/1
  ControlInput/1 -> State-Space (with initial outputs)/1
  Sum3/1 -> state/1, State4/1
  Matrix Multiply4/1 -> output/1, State3/1
  Constant2/1 -> Sum3/2

== system Control_Loop4_2Model/Plant2_Eq2 ==
  ControlInput : Inport  SampleTime=1
  Constant1 : Constant  Value=[1 0 0 0]  VectorParams1D=off  SampleTime=0.010
  Constant2 : Constant  Value=[-0.05;-0.05;-0.05;-0.05]  VectorParams1D=off  SampleTime=0.010
  Matrix Multiply1 : Product  Multiplication=Matrix(*)  SampleTime=0.010
  State-Space (with initial outputs) : simulink_extras/Additional Linear/State-Space (with initial outputs)  A=[0 1.0000 0 0;0 -2.6667 0.4000 0.6000;0 0 0 1.0000;0 2.0000 -0.4000 -0.6000]  B=[0;0.2667;0;-0.2000]  C=[1 0 0 0;0 1 0 0;0 0 1 0;0 0 0 1]  D=[0;0;0;0]  U0=0  Y0=1
  State3 : Scope
      settings: YMin=-0.5  YMax=1.1  SaveName=ScopeData45
  State4 : Scope
      settings: YMin=-0.07  YMax=0.08  SaveName=ScopeData46
  Sum : Sum  Inputs=|++
  state1 : Outport  SampleTime=1
  output1 : Outport  Port=2  SampleTime=1
  wires:
  State-Space (with initial outputs)/1 -> Sum/1, Matrix Multiply1/2
  Constant1/1 -> Matrix Multiply1/1
  ControlInput/1 -> State-Space (with initial outputs)/1
  Sum/1 -> State4/1, state1/1
  Matrix Multiply1/1 -> State3/1, output1/1
  Constant2/1 -> Sum/2

== system Control_Loop4_2Model/extractdec_F1 ==
  In1 : Inport
  ChangeVal : MATLAB Function  RequirementInfo={} %GIDa_56979559_068e_4e1b_8105_92ab20dfbbac  TreatAsAtomicUnit=on  SystemSampleTime=0.010
  Out1 : Outport
  Out2 : Outport  Port=2
  wires:
  ChangeVal/1(y1) -> Out1/1
  ChangeVal/2(y2) -> Out2/1
  In1/1 -> ChangeVal/1(u)

== system Control_Loop4_2Model/extractdec_F2 ==
  In1 : Inport
  ChangeVal : MATLAB Function  RequirementInfo={} %GIDa_1ad77da1_be0b_42ac_9201_349395f8b724  TreatAsAtomicUnit=on  SystemSampleTime=0.010
  Out1 : Outport
  Out2 : Outport  Port=2
  wires:
  ChangeVal/1(y1) -> Out1/1
  ChangeVal/2(y2) -> Out2/1
  In1/1 -> ChangeVal/1(u)

== system Control_Loop4_2Model/extractdec_F3 ==
  In1 : Inport
  ChangeVal : MATLAB Function  RequirementInfo={} %GIDa_f09461e8_b1c1_4233_9737_f1d9f81aa076  TreatAsAtomicUnit=on  SystemSampleTime=0.010
  Out1 : Outport
  Out2 : Outport  Port=2
  wires:
  ChangeVal/1(y1) -> Out1/1
  ChangeVal/2(y2) -> Out2/1
  In1/1 -> ChangeVal/1(u)

== system Control_Loop4_2Model/extractdec_F4 ==
  In1 : Inport
  ChangeVal : MATLAB Function  RequirementInfo={} %GIDa_db7bc024_9563_43a1_9102_360fc9c9ffae  TreatAsAtomicUnit=on  SystemSampleTime=0.010
  Out1 : Outport
  Out2 : Outport  Port=2
  wires:
  ChangeVal/1(y1) -> Out1/1
  ChangeVal/2(y2) -> Out2/1
  In1/1 -> ChangeVal/1(u)

== system Control_Loop4_2Model/extractdec_F5 ==
  In1 : Inport
  In2 : Inport  Port=2
  In3 : Inport  Port=3
  In4 : Inport  Port=4
  ChangeVal : MATLAB Function  RequirementInfo={} %GIDa_02dc1ce4_e52f_48c0_8d9f_2d2cba98e866  TreatAsAtomicUnit=on  SystemSampleTime=0.010
  Out1 : Outport
  Out2 : Outport  Port=2
  wires:
  ChangeVal/1(y1) -> Out1/1
  ChangeVal/2(y2) -> Out2/1
  In1/1 -> ChangeVal/1(u1)
  In2/1 -> ChangeVal/2(u2)
  In3/1 -> ChangeVal/3(u3)
  In4/1 -> ChangeVal/4(u4)

== system Control_Loop4_2Model/GISOO-Simulation Environment/CoojaConnector ==
  DelayNum. : Inport
  Check if Cooja is not at same time (behind) : RelationalOperator  Operator=>  OutDataTypeStr=boolean
  "Check that we don't loop forever, if Cooja never answers" : simulink/Logic and Bit Operations/Compare To Constant  relop=<  const=300000  OutDataTypeStr=uint8  ZeroCross=off
  Data Type Conversion1 : DataTypeConversion  OutDataTypeStr=uint32
  Digital Clock : DigitalClock  SampleTime=-1
  Mux : Mux  Inputs=3
  Mux5 : Mux  Inputs=16
  ReceiveFromCooja : xpclib/UDP/Receive  ipAddress=127.0.0.1  ipPort=55555  width=28  vblLen=off  sampletime=-1
  Stop : Assertion  AssertionFailFcn=No communication with Cooja;
  Terminator : Terminator
  Tolerance due to rounding errors : Bias
  Unpack : xpclib/UDP/Unpack  dimensions={[1],[1],[1],[1],[1],[1],[1],[1],[1],[1],[1],[1],[1],[1],[1],[1],[1],[1],[1]}  datatypes={'uint32','uint32','uint32','uint8','uint8','uint8','uint8','uint8','uint8','uint8','uint8','uint8','uint8','uint8','uint8','uint8','uint8','uint8','uint8'}  byteAlign=1
  to ms3 : Gain  Gain=1000  ParamDataTypeStr=uint32  OutDataTypeStr=Inherit: Inherit via back propagation
  Wait : Outport
  tag scope: A=global, SerialData=global
  wires:
  Unpack/19 -> Mux5/16
  Unpack/18 -> Mux5/15
  Unpack/17 -> Mux5/14
  Unpack/16 -> Mux5/13
  Unpack/15 -> Mux5/12
  Unpack/14 -> Mux5/11
  Unpack/13 -> Mux5/10
  Unpack/12 -> Mux5/9
  Unpack/11 -> Mux5/8
  Check if Cooja is not at same time (behind)/1 -> Data Type Conversion1/1, Wait/1
  Unpack/2 -> Mux/2  "MotePinID"
  Unpack/1 -> Tolerance due to rounding errors/1  "CoojaTime"
  Tolerance due to rounding errors/1 -> Check if Cooja is not at same time (behind)/2
  Unpack/3 -> Mux/3  "uValue"
  Data Type Conversion1/1 -> Mux/1
  "Check that we don't loop forever, if Cooja never answers"/1 -> Stop/1
  DelayNum./1 -> "Check that we don't loop forever, if Cooja never answers"/1
  Mux/1 -> [A]
  Mux5/1 -> [SerialData]
  Unpack/4 -> Mux5/1
  Unpack/5 -> Mux5/2
  Unpack/6 -> Mux5/3
  Unpack/7 -> Mux5/4
  Unpack/8 -> Mux5/5
  Unpack/9 -> Mux5/6
  Unpack/10 -> Mux5/7
  Digital Clock/1 -> to ms3/1
  ReceiveFromCooja/2 -> Terminator/1
  to ms3/1 -> Check if Cooja is not at same time (behind)/1
  ReceiveFromCooja/1 -> Unpack/1

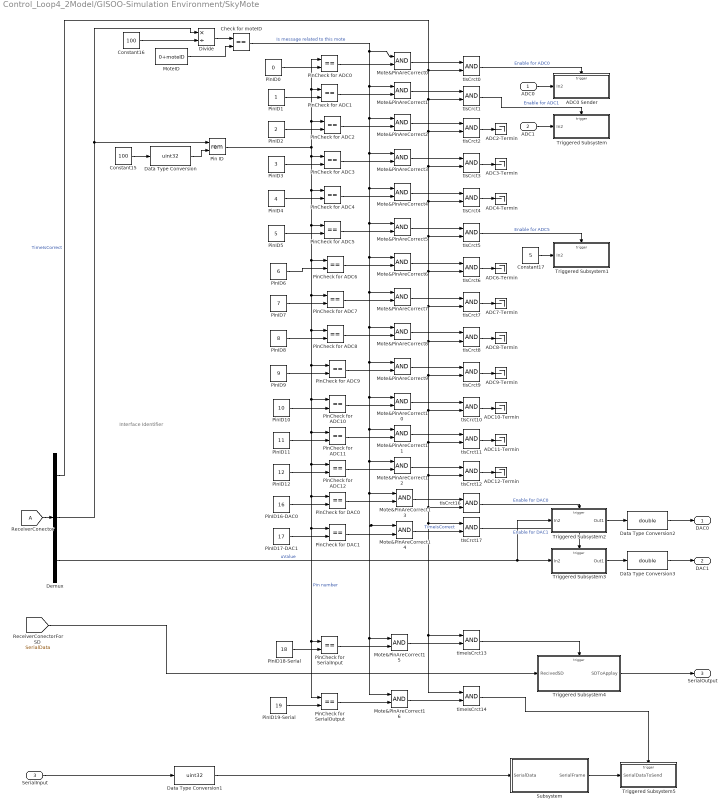
== system Control_Loop4_2Model/GISOO-Simulation Environment/SkyMote ==
  note: Interface Identifier
  ADC0 : Inport
  ADC1 : Inport  Port=2
  SerialInput : Inport  Port=3
  ADC0 Sender : Subsystem  TreatAsAtomicUnit=on
  ADC10-Termin : Terminator
  ADC11-Termin : Terminator
  ADC12-Termin : Terminator
  ADC2-Termin : Terminator
  ADC3-Termin : Terminator
  ADC4-Termin : Terminator
  ADC6-Termin : Terminator
  ADC7-Termin : Terminator
  ADC8-Termin : Terminator
  ADC9-Termin : Terminator
  Check for moteID : RelationalOperator  Operator===  OutDataTypeStr=boolean
  Constant15 : Constant  Value=100
  Constant16 : Constant  Value=100
  Constant17 : Constant  Value=5
  Data Type Conversion : DataTypeConversion  OutDataTypeStr=uint32
  Data Type Conversion1 : DataTypeConversion  OutDataTypeStr=uint32
  Data Type Conversion2 : DataTypeConversion  OutDataTypeStr=double
  Data Type Conversion3 : DataTypeConversion  OutDataTypeStr=double
  Demux : Demux  Outputs=3
  Divide : Product  Inputs=*/  OutDataTypeStr=int32
  Mote&PinAreCorrect{0..16} (17 alike) : Logic  AllPortsSameDT=off  OutDataTypeStr=boolean
  MoteID : Constant  Value=0+moteID
  Pin ID : Math  Operator=rem  SaturateOnIntegerOverflow=on
  PinCheck for ADC{0..12} (13 alike) : RelationalOperator  Operator===  OutDataTypeStr=boolean
  PinCheck for DAC0 : RelationalOperator  Operator===  OutDataTypeStr=boolean
  PinCheck for DAC1 : RelationalOperator  Operator===  OutDataTypeStr=boolean
  PinCheck for SerialInput : RelationalOperator  Operator===  OutDataTypeStr=boolean
  PinCheck for SerialOutput : RelationalOperator  Operator===  OutDataTypeStr=boolean
  PinID0 : Constant  Value=0
  PinID1 : Constant
  PinID10 : Constant  Value=10
  PinID11 : Constant  Value=11
  PinID12 : Constant  Value=12
  PinID16-DAC0 : Constant  Value=16
  PinID17-DAC1 : Constant  Value=17
  PinID18-Serial : Constant  Value=18
  PinID19-Serial : Constant  Value=19
  PinID2 : Constant  Value=2
  PinID3 : Constant  Value=3
  PinID4 : Constant  Value=4
  PinID5 : Constant  Value=5
  PinID6 : Constant  Value=6
  PinID7 : Constant  Value=7
  PinID8 : Constant  Value=8
  PinID9 : Constant  Value=9
  Subsystem : Subsystem
  Triggered Subsystem : Subsystem  TreatAsAtomicUnit=on
  Triggered Subsystem1 : Subsystem  TreatAsAtomicUnit=on
  Triggered Subsystem2 : Subsystem  TreatAsAtomicUnit=on
  Triggered Subsystem3 : Subsystem  TreatAsAtomicUnit=on
  Triggered Subsystem4 : Subsystem  TreatAsAtomicUnit=on
  Triggered Subsystem5 : Subsystem  TreatAsAtomicUnit=on
  tIsCrct{0..12,16..17} (15 alike) : Logic  AllPortsSameDT=off  OutDataTypeStr=boolean
  timeIsCrct13 : Logic  AllPortsSameDT=off  OutDataTypeStr=boolean
  timeIsCrct14 : Logic  AllPortsSameDT=off  OutDataTypeStr=boolean
  DAC0 : Outport
  DAC1 : Outport  Port=2
  SerialOutput : Outport  Port=3
  wires:
  Mote&PinAreCorrect11/1 -> tIsCrct11/1
  tIsCrct11/1 -> ADC11-Termin/1
  Mote&PinAreCorrect10/1 -> tIsCrct10/1
  tIsCrct10/1 -> ADC10-Termin/1
  Mote&PinAreCorrect9/1 -> tIsCrct9/1
  tIsCrct9/1 -> ADC9-Termin/1
  tIsCrct8/1 -> ADC8-Termin/1
  tIsCrct7/1 -> ADC7-Termin/1
  tIsCrct5/1 -> Triggered Subsystem1/Trigger  "Enable for ADC5"
  Mote&PinAreCorrect5/1 -> tIsCrct5/1
  tIsCrct6/1 -> ADC6-Termin/1
  tIsCrct4/1 -> ADC4-Termin/1
  tIsCrct3/1 -> ADC3-Termin/1
  Mote&PinAreCorrect2/1 -> tIsCrct2/1
  tIsCrct2/1 -> ADC2-Termin/1
  tIsCrct1/1 -> Triggered Subsystem/Trigger  "Enable for ADC1"
  Mote&PinAreCorrect1/1 -> tIsCrct1/1
  ADC1/1 -> Triggered Subsystem/1(In2)
  tIsCrct0/1 -> ADC0 Sender/Trigger  "Enable for ADC0"
  Mote&PinAreCorrect0/1 -> tIsCrct0/1
  Constant17/1 -> Triggered Subsystem1/1(In2)
  Triggered Subsystem3/1(Out1) -> Data Type Conversion3/1
  Data Type Conversion3/1 -> DAC1/1
  Triggered Subsystem2/1(Out1) -> Data Type Conversion2/1
  Data Type Conversion2/1 -> DAC0/1
  Demux/2 -> Pin ID/1, Divide/1
  ADC0/1 -> ADC0 Sender/1(In2)
  Demux/3 -> Triggered Subsystem2/1(In2), Triggered Subsystem3/1(In2)  "uValue"
  [A] -> Demux/1
  tIsCrct17/1 -> Triggered Subsystem3/Trigger  "Enable for DAC1"
  tIsCrct16/1 -> Triggered Subsystem2/Trigger  "Enable for DAC0"
  Data Type Conversion/1 -> Pin ID/2
  Constant15/1 -> Data Type Conversion/1
  Mote&PinAreCorrect3/1 -> tIsCrct3/1
  Mote&PinAreCorrect4/1 -> tIsCrct4/1
  Mote&PinAreCorrect6/1 -> tIsCrct6/1
  Mote&PinAreCorrect7/1 -> tIsCrct7/1
  Mote&PinAreCorrect8/1 -> tIsCrct8/1
  Mote&PinAreCorrect12/1 -> tIsCrct12/1
  Mote&PinAreCorrect13/1 -> tIsCrct16/1
  MoteID/1 -> Check for moteID/2
  Divide/1 -> Check for moteID/1
  Constant16/1 -> Divide/2
  PinCheck for DAC1/1 -> Mote&PinAreCorrect14/2
  PinCheck for DAC0/1 -> Mote&PinAreCorrect13/2
  PinCheck for ADC12/1 -> Mote&PinAreCorrect12/2
  PinCheck for ADC11/1 -> Mote&PinAreCorrect11/2
  PinCheck for ADC10/1 -> Mote&PinAreCorrect10/2
  PinCheck for ADC9/1 -> Mote&PinAreCorrect9/2
  PinCheck for ADC8/1 -> Mote&PinAreCorrect8/2
  PinCheck for ADC7/1 -> Mote&PinAreCorrect7/2
  PinCheck for ADC6/1 -> Mote&PinAreCorrect6/2
  PinCheck for ADC5/1 -> Mote&PinAreCorrect5/2
  PinCheck for ADC4/1 -> Mote&PinAreCorrect4/2
  PinCheck for ADC3/1 -> Mote&PinAreCorrect3/2
  PinCheck for ADC2/1 -> Mote&PinAreCorrect2/2
  PinCheck for ADC1/1 -> Mote&PinAreCorrect1/2
  PinCheck for ADC0/1 -> Mote&PinAreCorrect0/2
  PinID0/1 -> PinCheck for ADC0/2
  PinID2/1 -> PinCheck for ADC2/2
  PinID3/1 -> PinCheck for ADC3/2
  PinID4/1 -> PinCheck for ADC4/2
  PinID5/1 -> PinCheck for ADC5/2
  PinID6/1 -> PinCheck for ADC6/2
  PinID7/1 -> PinCheck for ADC7/2
  PinID8/1 -> PinCheck for ADC8/2
  PinID10/1 -> PinCheck for ADC10/2
  PinID1/1 -> PinCheck for ADC1/2
  PinID9/1 -> PinCheck for ADC9/2
  PinID11/1 -> PinCheck for ADC11/2
  PinID12/1 -> PinCheck for ADC12/2
  PinID16-DAC0/1 -> PinCheck for DAC0/2
  PinID17-DAC1/1 -> PinCheck for DAC1/2
  Subsystem/1(SerialFrame) -> Triggered Subsystem5/1(SerialDataToSend)
  Demux/1 -> tIsCrct0/2, tIsCrct1/2, tIsCrct2/2, tIsCrct3/2, tIsCrct4/2, tIsCrct5/2, tIsCrct6/2, tIsCrct7/2, tIsCrct8/2, tIsCrct9/2, tIsCrct10/2, tIsCrct11/2, tIsCrct12/2, tIsCrct16/2, timeIsCrct14/1, timeIsCrct13/1, tIsCrct17/1  "TimeIsCorrect"
  PinID18-Serial/1 -> PinCheck for SerialInput/2
  [SerialData] -> Triggered Subsystem4/1(RecivedSD)
  timeIsCrct13/1 -> Triggered Subsystem4/Trigger
  Mote&PinAreCorrect14/1 -> tIsCrct17/2  "TimeIsCorrect"
  Triggered Subsystem4/1(SDToApplay) -> SerialOutput/1
  tIsCrct12/1 -> ADC12-Termin/1
  Pin ID/1 -> PinCheck for ADC0/1, PinCheck for ADC1/1, PinCheck for ADC2/1, PinCheck for SerialOutput/1, PinCheck for SerialInput/1, PinCheck for DAC1/1, PinCheck for DAC0/1, PinCheck for ADC12/1, PinCheck for ADC11/1, PinCheck for ADC10/1, PinCheck for ADC9/1, PinCheck for ADC8/1, PinCheck for ADC7/1, PinCheck for ADC6/1, PinCheck for ADC5/1, PinCheck for ADC4/1, PinCheck for ADC3/1  "Pin number"
  Mote&PinAreCorrect15/1 -> timeIsCrct13/2
  Check for moteID/1 -> Mote&PinAreCorrect1/1, Mote&PinAreCorrect13/1, Mote&PinAreCorrect14/1, Mote&PinAreCorrect16/1, Mote&PinAreCorrect15/1, Mote&PinAreCorrect12/1, Mote&PinAreCorrect11/1, Mote&PinAreCorrect10/1, Mote&PinAreCorrect9/1, Mote&PinAreCorrect8/1, Mote&PinAreCorrect7/1, Mote&PinAreCorrect6/1, Mote&PinAreCorrect5/1, Mote&PinAreCorrect4/1, Mote&PinAreCorrect3/1, Mote&PinAreCorrect2/1, Mote&PinAreCorrect0/1  "Is message related to this mote"
  PinID19-Serial/1 -> PinCheck for SerialOutput/2
  PinCheck for SerialOutput/1 -> Mote&PinAreCorrect16/2
  Mote&PinAreCorrect16/1 -> timeIsCrct14/2
  timeIsCrct14/1 -> Triggered Subsystem5/Trigger
  SerialInput/1 -> Data Type Conversion1/1
  Data Type Conversion1/1 -> Subsystem/1(SerialData)
  PinCheck for SerialInput/1 -> Mote&PinAreCorrect15/2
